simulink model "SimulationDemo_Ship"  (R2025a)
settings: Solver=ode4  StartTime=0.0  StopTime=200  FixedStep=0.02  RelTol=1e-3
InitFcn:
  | Initialization
model workspace (MAT data in the model file):
  actuatorInitial.Aileron_deg = 0
  actuatorInitial.Elevator_deg = 0
  actuatorInitial.Rudder_deg = 0
  contactParams.Kz_Npm = 5000
  contactParams.Cz_Nspm = 160
  contactParams.FrictionMu = 0.03
  contactParams.SlipSpeed_mps = 0.15
  contactParams.RampGain_1pm = 200
  contactParams.NormalScaleMax = 8
  contactParams.GroundPitch_rad = 0.0523598775598
  contactParams.PitchK_NmPerRad = -0.5
  contactParams.PitchC_NmPerRadps = -1
  contactParams.LateralFrictionMu = 1.5
  contactParams.RollK_NmPerRad = -8
  contactParams.RollC_NmPerRadps = -2.5
  contactParams.YawK_NmPerRad = -12
  contactParams.YawC_NmPerRadps = -4
  flightProtection.VMin_mps = 2
  flightProtection.VEps_mps = 0.001
  flightProtection.QGateBreakpoints_mps = [0 2 5]
  flightProtection.QGateTable = [0 0 1]
  flightProtection.BetaGateStartU_mps = 8
  flightProtection.BetaGateFullU_mps = 18
  initial.Heading = -2.35619449019
  initial.Roll = 0
  initial.Pitch = 0.0523598775598
  initial.Yaw = -2.35619449019
  initial.p = 0
  initial.q = 0.0001
  initial.r = 0.0001
  initial.u = 0.1
  initial.v = 0
  initial.w = 0.001
  initial.Altitude_MSL = 0
  initial.Altitude_AGL = 0
  initial.CGInertial.X = 0
  initial.CGInertial.Y = 0
  initial.CGInertial.Z = 0
  initial.Xe = [0 0 0]
  initial.Mass.Empty = 1.67
  initial.Mass.Payload = 1.25
  initial.Mass.GrossTO = 2.92
  initial.Inertia = [0.026  0  0.0007; 0  0.072  0; 0.0007  0  0.096]
undefined symbols (not defined in the file): aeroData, aileronMax, aileronMin, dirPitch, dirRoll, dirThrottle, dirYaw, elevatorMax, elevatorMin, envCatalog, F, geometry, Light, MIL, pitchCh, pitchDB, propulsionData, rollCh, rollDB, rudderMax, rudderMin, throttleCh, throttleDB, uPitchMax, uPitchMin, uRollMax, uRollMin, uThrottleMax, uThrottleMin, uYawMax, uYawMin, yawCh, yawDB
libraries: simulink_extras x4, aerolibwind2 x3, aerolibasang x2, aerolibsim3d x2, aerolibadyn x1, matrix_library x1, aerolibanimutils x1, aerolibatmos2 x1, uavutilslib x1, sim3dlib x1
(part 1 of 2)
settings Model: DataDictionary=environmentData.sldd  Creator=klakhara  LastModifiedBy=klakhara
settings SolverCC: ODENIntegrationMethod=ode4

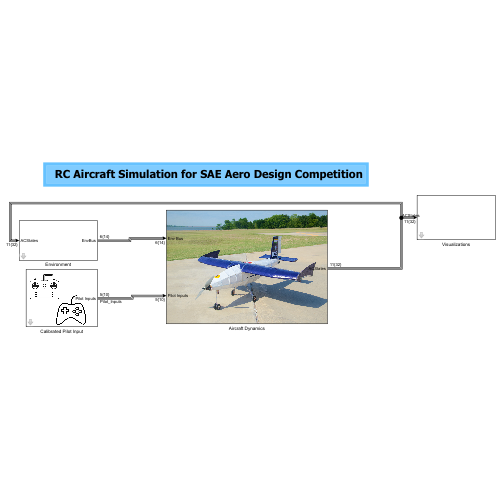
[thumbnail: Simulink's stored preview of the top-level diagram]
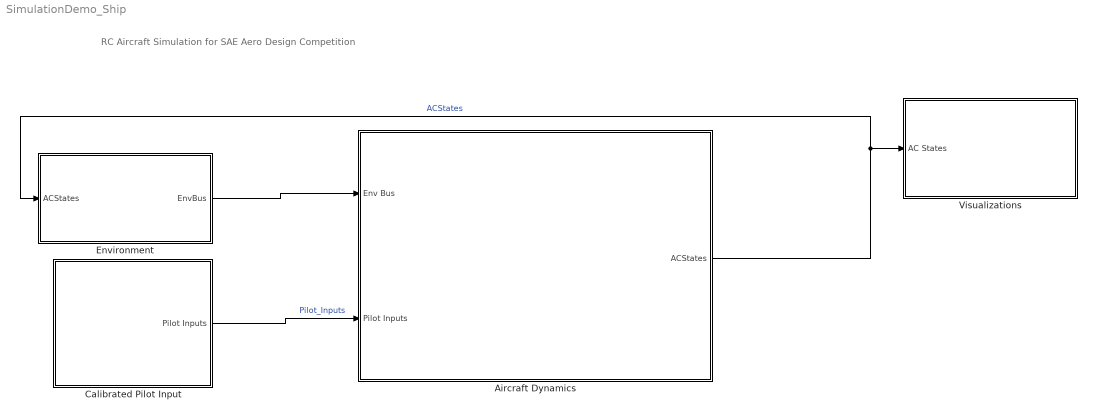
== system SimulationDemo_Ship ==
  note: RC Aircraft Simulation for SAE Aero Design Competition
  Aircraft Dynamics : Subsystem
      mask Display: image('Aircraft.jpg');
  Calibrated Pilot Input : Subsystem  mask{configName=0, joystickID=None}
      mask prompts: joystickID "Device ID:"
      mask TypeOptions joystickID: None | Joystick1 | Joystick2 | Joystick3 | Joystick4 | Joystick5 | Joystick6 | Joystick7 | Joystick8 | Joystick9 | Joystick10 | Joystick11 | Joystick12
      mask DialogControl DescGroupVar Prompt: Import calibration parameters to setup the calibreated input device
      mask DialogControl DescTextVar Prompt: Import your calibration configuration file:
      mask DialogControl loadConfig Prompt: Load file
      mask DialogControl ParameterGroupVar Prompt: Identify your Pilot Input Device:
      mask Display: image('Controller_Setup.jpg');
  Environment : Subsystem  mask{envPreset=Aero Design West — Van Nuys CA (1.1×)}
      mask prompts: envPreset "Select Environment scene"
      mask DialogControl Control1 Prompt: You can select among a variety of environment type along with their difficulty level.
  Visualizations : Subsystem  mask{visualization=Off, FlightParam=on}
      mask prompts: visualization "Trajectory visualization"; FlightParam "Plot flight parameters"
      mask DialogControl DescTextVar Prompt: Select your visualization type and if you want to plot flight paramets in scope.
      mask Display:
      | % Get selected variant from mask
      | v = get_param(gcb, 'visualization');
      | 
      | % Clear icon
      | cla;
      | 
      | 
      | % Choose image based on variant
      | switch v
      |     case '3D Animation'
      |         img = imread('3D_Animation.png');
      |         image(img);
      |         axis off
      |         axis image
      |     case "Unreal Engine"
      |         img = imread('Unreal_Engine.png');
      |         image(img);
      |         axis off
      |         axis image
      |     case 'Off'
      |         % No image
      | 
      | end
      | 
      | % Display image as block icon
  wires:
  Aircraft Dynamics/1(ACStates) -> Environment/1(ACStates), Visualizations/1(AC States)  "ACStates"
  Environment/1(EnvBus) -> Aircraft Dynamics/1(Env Bus)
  Calibrated Pilot Input/1(Pilot Inputs) -> Aircraft Dynamics/2(Pilot Inputs)  "Pilot_Inputs"

== system SimulationDemo_Ship/Aircraft Dynamics ==
  Env Bus : Inport
  Pilot Inputs : Inport  Port=2
  ACStates To Workspace : ToWorkspace  VariableName=ACStates  SaveFormat=Timeseries  SampleTime=-1
  Actuator Dynamics : Subsystem
  Bus Creator : BusCreator  Inputs=8
  Bus Selector : BusSelector  OutputSignals=Actuator deflections
  Equation of motion : EOM6DOFBodyQuat  xme_0=initial.Xe  Vm_0=[initial.u initial.v initial.w]  eul_0=[initial.Roll initial.Pitch initial.Yaw]  pm_0=[initial.p initial.q initial.r]  mass_0=initial.Mass.GrossTO  inertia=initial.Inertia
  Flight Parameters : Subsystem
  Forces & Moments : Subsystem
  Gain : Gain  Gain=[1, 1, -1]
  ACStates : Outport
  wires:
  Actuator Dynamics/1(Actuator_Deflections) -> Bus Creator/8, Forces & Moments/4(Pilot_Inputs)  "Actuator deflections"
  Bus Selector/1 -> Actuator Dynamics/1(Actuator_Command)  "<Actuator deflections>"
  Pilot Inputs/1 -> Bus Selector/1  "Pilot_Inputs"
  Forces & Moments/2(Moments) -> Equation of motion/2
  Forces & Moments/1(Forces) -> Equation of motion/1
  Flight Parameters/1(Flight_Parameters) -> Forces & Moments/2(Flight Params)
  Equation of motion/2 -> Gain/1
  Equation of motion/4 -> Bus Creator/4  "q"
  Gain/1 -> Bus Creator/2  "Xe"
  Env Bus/1 -> Flight Parameters/2(EnvirBus), Forces & Moments/3(Env Bus)
  Equation of motion/1 -> Bus Creator/1  "Ve"
  Equation of motion/5 -> Bus Creator/5  "DCM_be"
  Equation of motion/7 -> Bus Creator/7  "wb"
  Equation of motion/6 -> Bus Creator/6  "Vb"
  Equation of motion/3 -> Bus Creator/3  "Euler_angles"
  Bus Creator/1 -> Forces & Moments/1(States), Flight Parameters/1("AC States "), ACStates To Workspace/1, ACStates/1  "ACStates"

== system SimulationDemo_Ship/Calibrated Pilot Input ==
  Actuator scaling : Subsystem
  Bus Creator : BusCreator  Inputs=2
  Pilot Joystick All : aerolibanimutils/Pilot Joystick  JoystickID=None  OutputConfiguration=AllOutputs  SampleTime=0.5
  PilotInput : BusCreator  Inputs=4
  Terminator : Terminator
  Terminator1 : Terminator
  Pilot Inputs : Outport
  wires:
  Bus Creator/1 -> Pilot Inputs/1
  Pilot Joystick All/1 -> Bus Creator/1, Actuator scaling/1(In1)  "Raw Inputs"
  Actuator scaling/2(Elevator) -> PilotInput/2  "Elevator"
  Pilot Joystick All/2 -> Terminator/1
  PilotInput/1 -> Bus Creator/2  "Actuator deflections"
  Actuator scaling/3(Rudder) -> PilotInput/3  "Rudder"
  Actuator scaling/4(Throttle) -> PilotInput/4  "Throttle"
  Actuator scaling/1(Aileron) -> PilotInput/1  "Aileron"
  Pilot Joystick All/3 -> Terminator1/1

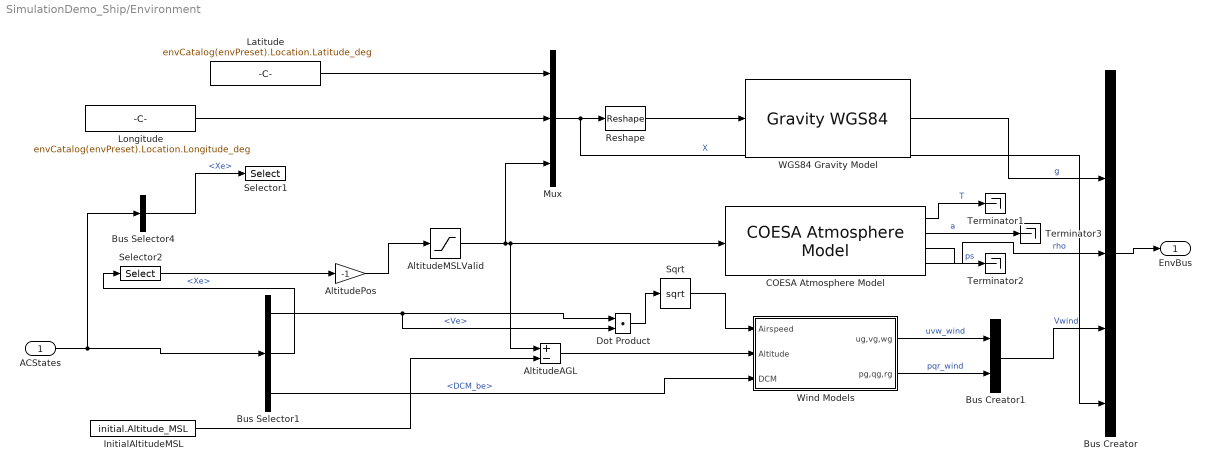
== system SimulationDemo_Ship/Environment ==
  ACStates : Inport
  AltitudeAGL : Sum  Inputs=+-
  AltitudeMSLValid : Saturate  UpperLimit=84852  LowerLimit=0
  AltitudePos : Gain  Gain=-1
  Bus Creator : BusCreator  Inputs=5
  Bus Creator1 : BusCreator  Inputs=2
  Bus Selector1 : BusSelector  OutputSignals=Ve,Xe,DCM_be
  Bus Selector4 : BusSelector  OutputSignals=Xe
  COESA Atmosphere Model : aerolibatmos2/COESA Atmosphere Model  units=Metric (MKS)  spec=1976 COESA-extended U.S. Standard Atmosphere  model=Profile  profile_var=High temperature  profile_percent=1%  profile_alt=5 km (16404 ft)  envelope_var=High temperature  envelope_percent=1%  action=Warning
  Dot Product : DotProduct  OutDataTypeStr=Inherit: Inherit via internal rule
  InitialAltitudeMSL : Constant  Value=initial.Altitude_MSL
  "Latitude " : Constant  Value=envCatalog(envPreset).Location.Latitude_deg
  Longitude : Constant  Value=envCatalog(envPreset).Location.Longitude_deg
  Mux : Mux  Inputs=3
  Reshape : Reshape  OutputDimensionality=Row vector (2-D)
  Selector1 : Selector  IndexMode=Zero-based  InputPortWidth=3  IndexOptions=Index vector (dialog)  Indices=2  OutputSizes=1
  Selector2 : Selector  IndexMode=Zero-based  InputPortWidth=3  IndexOptions=Index vector (dialog)  Indices=2  OutputSizes=1
  Sqrt : Sqrt
  Terminator1 : Terminator
  Terminator2 : Terminator
  Terminator3 : Terminator
  "WGS84 Gravity Model  " : GravityWGS84  action=None
  Wind Models : Subsystem
  EnvBus : Outport  VectorParamsAs1DForOutWhenUnconnected=off
  wires:
  AltitudeMSLValid/1 -> COESA Atmosphere Model/1, AltitudeAGL/1, Mux/3
  AltitudePos/1 -> AltitudeMSLValid/1
  AltitudeAGL/1 -> Wind Models/2(Altitude)
  InitialAltitudeMSL/1 -> AltitudeAGL/2
  Selector2/1 -> AltitudePos/1
  Bus Selector1/2 -> Selector2/1  "<Xe>"
  Bus Selector1/3 -> Wind Models/3(DCM)  "<DCM_be>"
  Reshape/1 -> "WGS84 Gravity Model  "/1
  "WGS84 Gravity Model  "/1 -> Bus Creator/2  "g"
  Mux/1 -> Reshape/1, Bus Creator/5  "X"
  Longitude/1 -> Mux/2
  "Latitude "/1 -> Mux/1
  Bus Selector1/1 -> Dot Product/1, Dot Product/2  "<Ve>"
  ACStates/1 -> Bus Selector4/1, Bus Selector1/1
  Bus Selector4/1 -> Selector1/1  "<Xe>"
  Bus Creator/1 -> EnvBus/1
  Sqrt/1 -> Wind Models/1(Airspeed)
  Dot Product/1 -> Sqrt/1
  Bus Creator1/1 -> Bus Creator/4  "Vwind"
  Wind Models/1(ug,vg,wg) -> Bus Creator1/1  "uvw_wind"
  Wind Models/2(pg,qg,rg) -> Bus Creator1/2  "pqr_wind"
  COESA Atmosphere Model/2 -> Terminator3/1  "a"
  COESA Atmosphere Model/3 -> Terminator2/1  "ps"
  COESA Atmosphere Model/1 -> Terminator1/1  "T"
  COESA Atmosphere Model/4 -> Bus Creator/3  "rho"

== system SimulationDemo_Ship/Visualizations ==
  AC States : Inport
  "Flight parameters " : Subsystem  Variant=on  EmptyChoice=on
  Trajectory Visualization : Subsystem  Variant=on  EmptyChoice=on
  wires:
  AC States/1 -> Trajectory Visualization/1(AC States), "Flight parameters "/1(In1)

== system SimulationDemo_Ship/Aircraft Dynamics/Actuator Dynamics ==
  Actuator_Command : Inport
  Aileron_Command_Limit : Saturate  UpperLimit=geometry.AileronLimit(2)  LowerLimit=geometry.AileronLimit(1)
  Aileron_Deflection_Limit : Saturate  UpperLimit=geometry.AileronLimit(2)  LowerLimit=geometry.AileronLimit(1)
  Aileron_Lag_0p05s : StateSpace  A=-20  B=20  D=0  InitialCondition=actuatorInitial.Aileron_deg
  Aileron_Rate_300dps : RateLimiter  RisingSlewLimit=300  FallingSlewLimit=-300  InitialCondition=actuatorInitial.Aileron_deg
  Command_Select : BusSelector  OutputSignals=Aileron,Elevator,Rudder,Throttle
  Deflection_Bus : BusCreator  Inputs=4
  Elevator_Command_Limit : Saturate  UpperLimit=geometry.ElevatorLimit(2)  LowerLimit=geometry.ElevatorLimit(1)
  Elevator_Deflection_Limit : Saturate  UpperLimit=geometry.ElevatorLimit(2)  LowerLimit=geometry.ElevatorLimit(1)
  Elevator_Lag_0p05s : StateSpace  A=-20  B=20  D=0  InitialCondition=actuatorInitial.Elevator_deg
  Elevator_Rate_300dps : RateLimiter  RisingSlewLimit=300  FallingSlewLimit=-300  InitialCondition=actuatorInitial.Elevator_deg
  Rudder_Command_Limit : Saturate  UpperLimit=geometry.RudderLimit(2)  LowerLimit=geometry.RudderLimit(1)
  Rudder_Deflection_Limit : Saturate  UpperLimit=geometry.RudderLimit(2)  LowerLimit=geometry.RudderLimit(1)
  Rudder_Lag_0p05s : StateSpace  A=-20  B=20  D=0  InitialCondition=actuatorInitial.Rudder_deg
  Rudder_Rate_300dps : RateLimiter  RisingSlewLimit=300  FallingSlewLimit=-300  InitialCondition=actuatorInitial.Rudder_deg
  Actuator_Deflections : Outport
  wires:
  Actuator_Command/1 -> Command_Select/1
  Aileron_Command_Limit/1 -> Aileron_Lag_0p05s/1
  Command_Select/1 -> Aileron_Command_Limit/1  "<Aileron>"
  Command_Select/2 -> Elevator_Command_Limit/1  "<Elevator>"
  Command_Select/3 -> Rudder_Command_Limit/1  "<Rudder>"
  Elevator_Command_Limit/1 -> Elevator_Lag_0p05s/1
  Command_Select/4 -> Deflection_Bus/4  "<Throttle>"
  Rudder_Command_Limit/1 -> Rudder_Lag_0p05s/1
  Aileron_Lag_0p05s/1 -> Aileron_Rate_300dps/1
  Elevator_Lag_0p05s/1 -> Elevator_Rate_300dps/1
  Rudder_Lag_0p05s/1 -> Rudder_Rate_300dps/1
  Aileron_Rate_300dps/1 -> Aileron_Deflection_Limit/1
  Elevator_Rate_300dps/1 -> Elevator_Deflection_Limit/1
  Rudder_Rate_300dps/1 -> Rudder_Deflection_Limit/1
  Elevator_Deflection_Limit/1 -> Deflection_Bus/2  "Elevator"
  Aileron_Deflection_Limit/1 -> Deflection_Bus/1  "Aileron"
  Rudder_Deflection_Limit/1 -> Deflection_Bus/3  "Rudder"
  Deflection_Bus/1 -> Actuator_Deflections/1

== system SimulationDemo_Ship/Aircraft Dynamics/Flight Parameters ==
  "AC States " : Inport
  EnvirBus : Inport  Port=2
  Bus Creator : BusCreator  Inputs=6
  Bus Selector1 : BusSelector  OutputSignals=rho
  Bus Selector2 : BusSelector  OutputSignals=Vb
  Bus Selector3 : BusSelector  OutputSignals=wb
  Bus Selector4 : BusSelector  OutputSignals=Vwind.uvw_wind,Vwind.pqr_wind
  Flight Parameters To Workspace : ToWorkspace  VariableName=FlightParameters  SaveFormat=Timeseries  SampleTime=-1
  "Incidence, Sideslip, & Airspeed" : aerolibasang/Incidence, Sideslip, & Airspeed
  Radians to Degrees : simulink_extras/Transformations/Radians to Degrees
  Radians to Degrees1 : simulink_extras/Transformations/Radians to Degrees
  Subsystem : Subsystem
      settings: PortSchema="{\"entries\":[{\"content\":{\"sides\":[{\"content\":{\"connectorIds\":[\"In1\",\"In2\"]},\"type\":\"ConnectorPlacement.EquallySpacedRectSide\",\"uuid\":\"5a143d0f-2436-4fb0-bb97-2c4984d07975\"},{\"content\":{\"connectorIds\":[\"Out1\"],\"side\":\"RIGHT\"},\"type\":\"ConnectorPlacement.EquallySpacedRectSide\",\"uuid\":\"8d58a2ee-82c7-4615-9bab-8cc4c0d46ad5\"},{\"content\":{\"connectorIds\":[\"In3\"],\"side\":\"TOP\"},\"type\":\"ConnectorPlacement.EquallySpacedRectSide\",\"uuid\":\"18f756c1-07a2-4df5-83f0-d5c22876817a\"}]},\"type\":\"ConnectorPlacement.EquallySpacedConnector\",\"uuid\":\"42d60932-45cf-443a-a7ca-3ff9305e2569\"}],\"packageUris\":[\"http://schema.mathworks.com/mf0/Connector/R2020b\"],\"version\":\"1.0\"}"
  Sum2 : Sum  InputSameDT=on  SaturateOnIntegerOverflow=on  OutDataTypeStr=Inherit: Same as first input
  Sum4 : Sum  Inputs=+-|  InputSameDT=on  SaturateOnIntegerOverflow=on  OutDataTypeStr=Inherit: Same as first input
  Vrel_safe : Subsystem
  Flight_Parameters : Outport  VectorParamsAs1DForOutWhenUnconnected=off
  wires:
  "AC States "/1 -> Bus Selector2/1, Bus Selector3/1
  Sum2/1 -> Bus Creator/5  "pqr_tot"
  Sum4/1 -> Vrel_safe/1(Vrel)  "Vrel"
  Bus Selector3/1 -> Sum2/2  "<wb>"
  EnvirBus/1 -> Bus Selector1/1, Bus Selector4/1
  Bus Selector2/1 -> Sum4/1  "<Vb>"
  Bus Selector4/2 -> Sum2/1  "<pqr_wind>"
  Bus Selector4/1 -> Sum4/2  "<uvw_wind>"
  "Incidence, Sideslip, & Airspeed"/3 -> Subsystem/3(TAS), Bus Creator/4  "TAS"
  "Incidence, Sideslip, & Airspeed"/1 -> Radians to Degrees/1
  "Incidence, Sideslip, & Airspeed"/2 -> Radians to Degrees1/1
  Vrel_safe/1(Vrel_safe) -> Subsystem/1(Vrel_safe), "Incidence, Sideslip, & Airspeed"/1, Bus Creator/1  "Vrel"
  Bus Selector1/1 -> Subsystem/2(<rho>)  "<rho>"
  Subsystem/1(q) -> Bus Creator/6  "dynamic Pressure"
  Radians to Degrees/1 -> Bus Creator/2  "alpha"
  Radians to Degrees1/1 -> Bus Creator/3  "beta"
  Bus Creator/1 -> Flight Parameters To Workspace/1, Flight_Parameters/1

== system SimulationDemo_Ship/Aircraft Dynamics/Forces & Moments ==
  note: Forces & Moments
      | 1. Gravitational Forces
      | 2. Aerodynamic Forces & Moments
      | 3. Propulsion Forces & Moments
  States : Inport
  Flight Params : Inport  Port=2
  Env Bus : Inport  Port=3
  Pilot_Inputs : Inport  Port=4
  Aerodynamic Forces & Moments : Subsystem
  Bus Selector : BusSelector  OutputSignals=g
  Bus Selector1 : BusSelector  OutputSignals=Xe,DCM_be,Vb
  Contact Forces & Moments : Subsystem
  Gravitational Forces : Subsystem
  Propulsion Forces & Moments : Subsystem
  Sum : Sum  Inputs=++++
  Sum1 : Sum  Inputs=+++
  Forces : Outport
  Moments : Outport  Port=2
  wires:
  Bus Selector1/3 -> Contact Forces & Moments/4(Vb)  "<Vb>"
  Contact Forces & Moments/1(F_Contact) -> Sum/4
  Bus Selector1/1 -> Contact Forces & Moments/2(Xe)  "<Xe>"
  Bus Selector1/2 -> Gravitational Forces/1(DCM)  "<DCM_be>"
  Sum1/1 -> Moments/1  "Moments"
  Sum/1 -> Forces/1  "Forces"
  Propulsion Forces & Moments/1(Forces_Propulsion) -> Sum/3  "F_Prop"
  Aerodynamic Forces & Moments/1(Forces_aero) -> Sum/2  "F_Aero"
  Gravitational Forces/1(Fgrav) -> Sum/1, Contact Forces & Moments/3(F_Gravity)  "F_Gravity"
  Bus Selector/1 -> Gravitational Forces/2(g)  "<g>"
  States/1 -> Bus Selector1/1, Contact Forces & Moments/1(States)  "States"
  Env Bus/1 -> Propulsion Forces & Moments/2(EnvBus), Bus Selector/1
  Flight Params/1 -> Aerodynamic Forces & Moments/1(Flight Params)
  Propulsion Forces & Moments/2(Moments_Propulsion) -> Sum1/2  "M_Prop"
  Pilot_Inputs/1 -> Aerodynamic Forces & Moments/2(Pilot_Input), Propulsion Forces & Moments/1(Pilot Inputs)
  Aerodynamic Forces & Moments/2(Moments_aero) -> Sum1/1  "M_Aero"
  Contact Forces & Moments/2(M_Contact) -> Sum1/3  "M_Contact"

== system SimulationDemo_Ship/Calibrated Pilot Input/Actuator scaling ==
  In1 : Inport
  Aileron Scaling : Subsystem
  Demux : Demux
  Elevator Scaling : Subsystem
  Rudder Scaling : Subsystem
  Selector : Selector  InputPortWidth=6  IndexOptions=Index vector (dialog)  Indices=[rollCh pitchCh yawCh throttleCh]  OutputSizes=1
  Throttle Scaling : Subsystem
  Aileron : Outport
  Elevator : Outport  Port=2
  Rudder : Outport  Port=3
  Throttle : Outport  Port=4
  wires:
  In1/1 -> Selector/1
  Rudder Scaling/1(actuator deflection) -> Rudder/1
  Demux/3 -> Rudder Scaling/1(raw signal)  "Yaw"
  Demux/1 -> Aileron Scaling/1(raw signal)  "roll"
  Elevator Scaling/1(actuator deflection) -> Elevator/1
  Demux/4 -> Throttle Scaling/1(raw signal)  "Throttle"
  Demux/2 -> Elevator Scaling/1(raw signal)  "Pitch"
  Aileron Scaling/1(actuator deflection) -> Aileron/1
  Throttle Scaling/1(actuator deflection) -> Throttle/1
  Selector/1 -> Demux/1

== system SimulationDemo_Ship/Environment/Wind Models ==
  Airspeed : Inport  Unit=m/s
  Altitude : Inport  Port=2  Unit=meter
  DCM : Inport  Port=3
  "DCM " : InportShadow  Port=3
  Discrete Wind Gust Model : aerolibwind2/Discrete Wind Gust Model  units=Metric (MKS)  Gx=off  Gy=off  Gz=off  t_0=envCatalog(envPreset).Gust.StartTime_s  d_m=envCatalog(envPreset).Gust.Length_m  v_m=envCatalog(envPreset).Gust.Amplitude_mps
  Dryden Wind Turbulence Model (Continuous (+q -r)) : aerolibwind2/Dryden Wind Turbulence Model  (Continuous (+q -r))  units=Metric (MKS)  spec=MIL-F-8785C  model=Continuous Dryden (+q -r)  W20=envCatalog(envPreset).Turbulence.Speed_6m_mps  Wdeg=envCatalog(envPreset).Turbulence.Direction_deg  TurbProb=10^-2 - Light  L_high=envCatalog(envPreset).Turbulence.Scale_Lu_m  Wingspan=geometry.Area  ts=0.5  Seed=envCatalog(envPreset).Turbulence.NoiseSeeds  T_on=off
  Sum : Sum  Inputs=+++  InputSameDT=on  SaturateOnIntegerOverflow=on  OutDataTypeStr=Inherit: Same as first input
  Wind Shear Model : aerolibwind2/Wind Shear Model  units=Metric (MKS)  phase=Category C - Terminal Flight Phase  W_20=envCatalog(envPreset).WindShear.Speed_6m_mps  Wdeg=envCatalog(envPreset).WindShear.Direction_deg
  ug,vg,wg : Outport  Unit=m/s  VectorParamsAs1DForOutWhenUnconnected=off
  pg,qg,rg : Outport  Port=2  Unit=rad/second  VectorParamsAs1DForOutWhenUnconnected=off
  wires:
  "DCM "/1 -> Dryden Wind Turbulence Model (Continuous (+q -r))/3
  Wind Shear Model/1 -> Sum/1
  Dryden Wind Turbulence Model (Continuous (+q -r))/1 -> Sum/2
  Discrete Wind Gust Model/1 -> Sum/3
  Sum/1 -> ug,vg,wg/1
  DCM/1 -> Wind Shear Model/2
  Airspeed/1 -> Dryden Wind Turbulence Model (Continuous (+q -r))/2, Discrete Wind Gust Model/1
  Dryden Wind Turbulence Model (Continuous (+q -r))/2 -> pg,qg,rg/1
  Altitude/1 -> Dryden Wind Turbulence Model (Continuous (+q -r))/1, Wind Shear Model/1

== system SimulationDemo_Ship/Visualizations/Flight parameters  ==
  In1 : Inport
  Scope Plot : Subsystem  TreatAsAtomicUnit=on  VariantControl=FlightParam ==1

== system SimulationDemo_Ship/Visualizations/Trajectory Visualization ==
  AC States : Inport
  3D Animation : Subsystem  VariantControl="visualization == \"3D Animation\""
      mask Display: image('3D_Animation.png');
  Unreal Engine : Subsystem  VariantControl="visualization == \"Unreal Engine\""
      mask Display: image('Unreal_Engine.png');

== system SimulationDemo_Ship/Aircraft Dynamics/Flight Parameters/Subsystem ==
  note: Note: 1D lookup table here is used as a switch to protect dynamic pressure for speed below 2 m/sec and gradually ramps up till 5 m/sec.
  Vrel_safe : Inport
  <rho> : Inport  Port=2
  TAS : Inport  Port=3
  1-D Lookup Table : Lookup_n-D  NumberOfTableDimensions=1  BreakpointsForDimension1=flightProtection.QGateBreakpoints_mps  Table=flightProtection.QGateTable  InterpMethod=Flat  ExtrapMethod=Clip  InternalRulePriority=Speed  RndMeth=Simplest
  Dynamic Pressure : aerolibasang/Dynamic Pressure
  Product : Product
  q : Outport
  wires:
  Vrel_safe/1 -> Dynamic Pressure/1
  <rho>/1 -> Dynamic Pressure/2
  1-D Lookup Table/1 -> Product/1
  Dynamic Pressure/1 -> Product/2
  Product/1 -> q/1
  TAS/1 -> 1-D Lookup Table/1

== system SimulationDemo_Ship/Aircraft Dynamics/Flight Parameters/Vrel_safe ==
  Vrel : Inport
  Mux_Vrel_safe : Mux  Inputs=3
  Split_Vrel : Demux  Outputs=3
  V_denom : MinMax  Function=max  Inputs=2
  V_min : Constant  Value=flightProtection.VMin_mps
  V_safe : MinMax  Function=max  Inputs=2
  eps_V : Constant  Value=flightProtection.VEps_mps
  scale : Product  Inputs=*/
  speed_sq : Sum  Inputs=+++
  sqrt_speed : Math  Operator=sqrt  SignedPower=on  RndMeth=Zero
  u_safe : Product
  u_sq : Product
  v_safe : Product
  v_sq : Product
  w_safe : Product
  w_sq : Product
  Vrel_safe : Outport
  wires:
  speed_sq/1 -> sqrt_speed/1  "V_mag_sq"
  Vrel/1 -> Split_Vrel/1
  u_sq/1 -> speed_sq/1
  w_sq/1 -> speed_sq/3
  Split_Vrel/1 -> u_sq/2, u_sq/1, u_safe/1  "u_rel"
  Split_Vrel/2 -> v_sq/1, v_sq/2, v_safe/1  "v_rel"
  v_sq/1 -> speed_sq/2
  Split_Vrel/3 -> w_safe/1, w_sq/2, w_sq/1  "w_rel"
  V_min/1 -> V_safe/2
  sqrt_speed/1 -> V_safe/1, V_denom/1  "V_mag"
  eps_V/1 -> V_denom/2
  V_safe/1 -> scale/1  "V_safe_mag"
  V_denom/1 -> scale/2
  u_safe/1 -> Mux_Vrel_safe/1  "u_rel_safe"
  scale/1 -> v_safe/2, w_safe/2, u_safe/2  "V_guard_scale"
  w_safe/1 -> Mux_Vrel_safe/3  "w_rel_safe"
  v_safe/1 -> Mux_Vrel_safe/2  "v_rel_safe"
  Mux_Vrel_safe/1 -> Vrel_safe/1  "Vrel_safe"

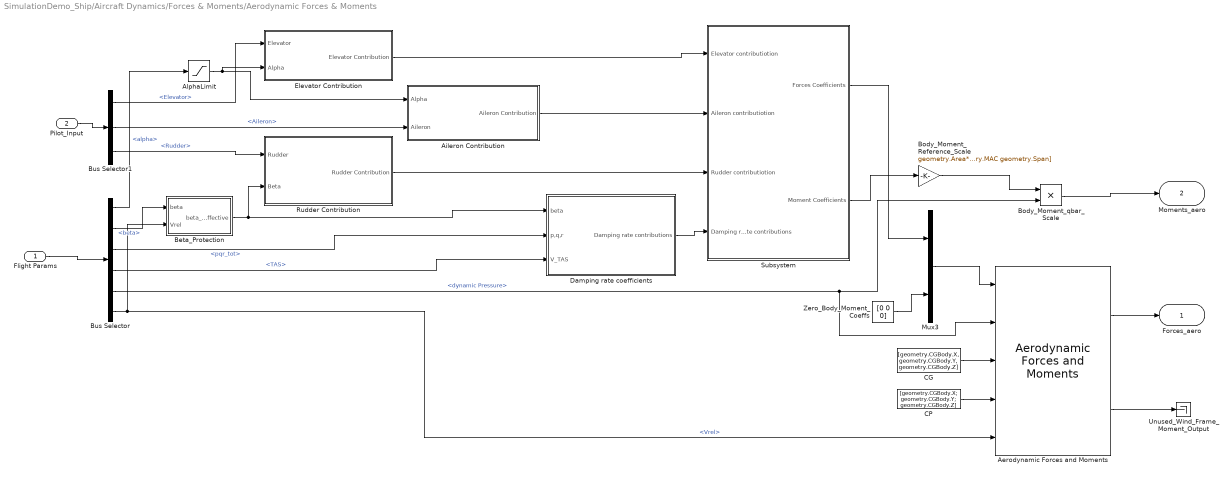
== system SimulationDemo_Ship/Aircraft Dynamics/Forces & Moments/Aerodynamic Forces & Moments ==
  Flight Params : Inport
  Pilot_Input : Inport  Port=2
  "Aerodynamic Forces and Moments " : aerolibadyn/Aerodynamic Forces and Moments   inputAxes=Wind  outputForceAxes=Body  outputMomentAxes=Body  S=geometry.Area  b=geometry.Span  cbar=geometry.MAC
  Aileron Contribution : Subsystem
  AlphaLimit : Saturate  UpperLimit=aeroData.validAlphaRange_deg(2)  LowerLimit=aeroData.validAlphaRange_deg(1)
  Beta_Protection : Subsystem
  Body_Moment_Reference_Scale : Gain  Gain=geometry.Area*[geometry.Span geometry.MAC geometry.Span]
  Body_Moment_qbar_Scale : Product
  Bus Selector : BusSelector  OutputSignals=alpha,beta,pqr_tot,TAS,dynamic Pressure,Vrel
  Bus Selector1 : BusSelector  OutputSignals=Elevator,Aileron,Rudder
  CG : Constant  Value="[geometry.CGBody.X, geometry.CGBody.Y,  geometry.CGBody.Z]"
  CP : Constant  Value=[geometry.CGBody.X; geometry.CGBody.Y; geometry.CGBody.Z]
  Damping rate coefficients : Subsystem
  Elevator Contribution : Subsystem
  Mux3 : Mux  Inputs=2
  Rudder Contribution : Subsystem
  Subsystem : Subsystem
  Unused_Wind_Frame_Moment_Output : Terminator
  Zero_Body_Moment_Coeffs : Constant  Value=[0 0 0]
  Forces_aero : Outport
  Moments_aero : Outport  Port=2
  wires:
  "Aerodynamic Forces and Moments "/2 -> Unused_Wind_Frame_Moment_Output/1
  Bus Selector/1 -> AlphaLimit/1  "<alpha>"
  Flight Params/1 -> Bus Selector/1
  Bus Selector/4 -> Damping rate coefficients/3(V_TAS)  "<TAS>"
  AlphaLimit/1 -> Elevator Contribution/2(Alpha), Aileron Contribution/1(Alpha)
  Bus Selector/2 -> Beta_Protection/1(beta)  "<beta>"
  Bus Selector/3 -> Damping rate coefficients/2(p,q,r)  "<pqr_tot>"
  Elevator Contribution/1(Elevator Contribution) -> Subsystem/1(Elevator contributiotion)
  Bus Selector/5 -> Body_Moment_qbar_Scale/2, "Aerodynamic Forces and Moments "/2  "<dynamic Pressure>"
  Bus Selector/6 -> Beta_Protection/2(Vrel), "Aerodynamic Forces and Moments "/5  "<Vrel>"
  CG/1 -> "Aerodynamic Forces and Moments "/3
  CP/1 -> "Aerodynamic Forces and Moments "/4
  Pilot_Input/1 -> Bus Selector1/1
  Bus Selector1/1 -> Elevator Contribution/1(Elevator)  "<Elevator>"
  Bus Selector1/2 -> Aileron Contribution/2(Aileron)  "<Aileron>"
  Bus Selector1/3 -> Rudder Contribution/1(Rudder)  "<Rudder>"
  Aileron Contribution/1(Aileron Contribution) -> Subsystem/2(Aileron contributiotion)
  Rudder Contribution/1("Rudder Contribution ") -> Subsystem/3(Rudder contributiotion)
  Damping rate coefficients/1(Damping rate contributions) -> Subsystem/4(Damping rate contributions)
  Subsystem/1(Forces Coefficients) -> Mux3/1
  Mux3/1 -> "Aerodynamic Forces and Moments "/1
  "Aerodynamic Forces and Moments "/1 -> Forces_aero/1
  Beta_Protection/1(beta_effective) -> Damping rate coefficients/1(beta), Rudder Contribution/2(Beta)
  Zero_Body_Moment_Coeffs/1 -> Mux3/2
  Subsystem/2(Moment Coefficients) -> Body_Moment_Reference_Scale/1
  Body_Moment_Reference_Scale/1 -> Body_Moment_qbar_Scale/1
  Body_Moment_qbar_Scale/1 -> Moments_aero/1

== system SimulationDemo_Ship/Aircraft Dynamics/Forces & Moments/Contact Forces & Moments ==
  States : Inport
  Xe : Inport  Port=2
  F_Gravity : Inport  Port=3
  Vb : Inport  Port=4
  Contact_Force_Total : Sum
  Ground_Contact_Switch : Switch  Criteria=u2 > Threshold  Threshold=initial.Mass.GrossTO*9.80665/contactParams.Kz_Npm
  Normal_Friction_Forces : Subsystem
  Pitch_Contact_Moment : Subsystem
  Select_Ze : Selector  InputPortWidth=3  IndexOptions=Index vector (dialog)  Indices=[3]  OutputSizes=1
  Zero_Force : Constant  Value=[0;0;0]
  F_Contact : Outport
  M_Contact : Outport  Port=2
  wires:
  Pitch_Contact_Moment/1(M_Contact) -> M_Contact/1  "M_Contact"
  States/1 -> Normal_Friction_Forces/4(States), Pitch_Contact_Moment/1(States)
  Normal_Friction_Forces/2(F_Contact_Friction) -> Contact_Force_Total/2
  Normal_Friction_Forces/1(F_Contact_Normal) -> Contact_Force_Total/1
  Vb/1 -> Normal_Friction_Forces/3(Vb)
  F_Gravity/1 -> Normal_Friction_Forces/2(F_Gravity)
  Contact_Force_Total/1 -> Ground_Contact_Switch/3
  Ground_Contact_Switch/1 -> F_Contact/1
  Zero_Force/1 -> Ground_Contact_Switch/1
  Select_Ze/1 -> Normal_Friction_Forces/1(Ze), Ground_Contact_Switch/2
  Xe/1 -> Select_Ze/1

== system SimulationDemo_Ship/Aircraft Dynamics/Forces & Moments/Gravitational Forces ==
  DCM : Inport
  g : Inport  Port=2  Unit=m/s^2
  Gross TO mass : Gain  Gain=initial.Mass.GrossTO  SaturateOnIntegerOverflow=on  OutDataTypeStr=Inherit: Same as input  ParamDataTypeStr=Inherit: Same as input
  Inertial to Body : Product  Multiplication=Matrix(*)  InputSameDT=on  SaturateOnIntegerOverflow=on  OutDataTypeStr=Inherit: Same as first input
  Reshape : Reshape  OutputDimensionality=Column vector (2-D)
  Reshape1 : Reshape
  Fgrav : Outport  Unit=N  VectorParamsAs1DForOutWhenUnconnected=off
  wires:
  Inertial to Body/1 -> Reshape1/1
  g/1 -> Gross TO mass/1
  DCM/1 -> Inertial to Body/1
  Gross TO mass/1 -> Reshape/1
  Reshape/1 -> Inertial to Body/2
  Reshape1/1 -> Fgrav/1

== system SimulationDemo_Ship/Aircraft Dynamics/Forces & Moments/Propulsion Forces & Moments ==
  Pilot Inputs : Inport
  EnvBus : Inport  Port=2
  Density Correction : Subsystem
  Gain : Gain
  Product : Product
  Subsystem : Subsystem
      settings: PortSchema="{\"entries\":[{\"content\":{\"sides\":[{\"content\":{\"connectorIds\":[\"Out1\"]},\"type\":\"ConnectorPlacement.EquallySpacedRectSide\",\"uuid\":\"fb30b856-b505-4c52-9be5-f51b9b4f9b3d\"},{\"content\":{\"side\":\"RIGHT\"},\"type\":\"ConnectorPlacement.EquallySpacedRectSide\",\"uuid\":\"6b49ea0c-e042-48c7-9a23-d0c81f552445\"},{\"content\":{\"connectorIds\":[\"In1\"],\"side\":\"TOP\"},\"type\":\"ConnectorPlacement.EquallySpacedRectSide\",\"uuid\":\"9dc7e958-cdfa-43a2-9a4f-607dc953e274\"}]},\"type\":\"ConnectorPlacement.EquallySpacedConnector\",\"uuid\":\"2adf19d2-e141-4d29-811e-0d4bf7e85bad\"}],\"packageUris\":[\"http://schema.mathworks.com/mf0/Connector/R2020b\"],\"version\":\"1.0\"}"
  Subsystem1 : Subsystem
  Subsystem2 : Subsystem
  Forces_Propulsion : Outport
  Moments_Propulsion : Outport  Port=2
  wires:
  Gain/1 -> Forces_Propulsion/1, Subsystem/1(Forces)
  Product/1 -> Subsystem1/1(Density corrected Thrust)
  Subsystem1/1(Forces_Propulsion) -> Gain/1
  Subsystem/1(Moments) -> Moments_Propulsion/1  "Moments_Propulsion"
  EnvBus/1 -> Density Correction/1(In1)
  Density Correction/1(Out1) -> Product/2
  Pilot Inputs/1 -> Subsystem2/1(Pilot_Inputs)  "Pilot_Inputs"
  Subsystem2/1(Motor_Prop_Thrust) -> Product/1

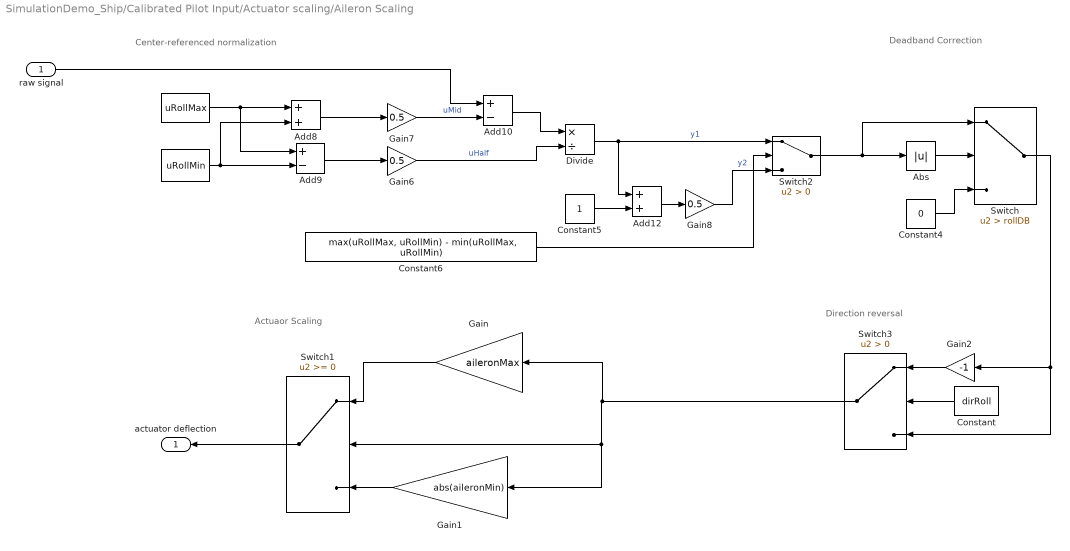
== system SimulationDemo_Ship/Calibrated Pilot Input/Actuator scaling/Aileron Scaling ==
  note: Direction reversal
  note: Center-referenced normalization
  note: Deadband Correction
  note: Actuaor Scaling
  raw signal : Inport
  " " : Constant  Value=uRollMin
  "   " : Constant  Value=uRollMax
  Abs : Abs  SaturateOnIntegerOverflow=off
  Add10 : Sum  Inputs=+-
  Add12 : Sum
  Add8 : Sum
  Add9 : Sum  Inputs=+-
  Constant : Constant  Value=dirRoll
  Constant4 : Constant  Value=0
  Constant5 : Constant
  Constant6 : Constant  Value=max(uRollMax, uRollMin) - min(uRollMax, uRollMin)
  Divide : Product  Inputs=*/
  Gain : Gain  Gain=aileronMax
  Gain1 : Gain  Gain=abs(aileronMin)
  Gain2 : Gain  Gain=-1
  Gain6 : Gain  Gain=0.5
  Gain7 : Gain  Gain=0.5
  Gain8 : Gain  Gain=0.5
  Switch : Switch  Criteria=u2 > Threshold  Threshold=rollDB  SaturateOnIntegerOverflow=off  InputSameDT=off
  Switch1 : Switch  SaturateOnIntegerOverflow=off  InputSameDT=off
  Switch2 : Switch  Criteria=u2 > Threshold  SaturateOnIntegerOverflow=off  InputSameDT=off
  Switch3 : Switch  Criteria=u2 > Threshold  SaturateOnIntegerOverflow=off  InputSameDT=off
  actuator deflection : Outport
  wires:
  Add9/1 -> Gain6/1
  "   "/1 -> Add9/1, Add8/1
  Add8/1 -> Gain7/1
  " "/1 -> Add8/2, Add9/2
  raw signal/1 -> Add10/1
  Gain7/1 -> Add10/2  "uMid"
  Add10/1 -> Divide/1
  Gain6/1 -> Divide/2  "uHalf"
  Switch1/1 -> actuator deflection/1
  Divide/1 -> Add12/1, Switch2/1  "y1"
  Constant5/1 -> Add12/2
  Add12/1 -> Gain8/1
  Constant6/1 -> Switch2/2
  Gain8/1 -> Switch2/3  "y2"
  Abs/1 -> Switch/2
  Constant4/1 -> Switch/3
  Switch/1 -> Gain2/1, Switch3/3
  Gain/1 -> Switch1/1
  Gain1/1 -> Switch1/3
  Gain2/1 -> Switch3/1
  Switch3/1 -> Gain1/1, Switch1/2, Gain/1
  Constant/1 -> Switch3/2
  Switch2/1 -> Switch/1, Abs/1

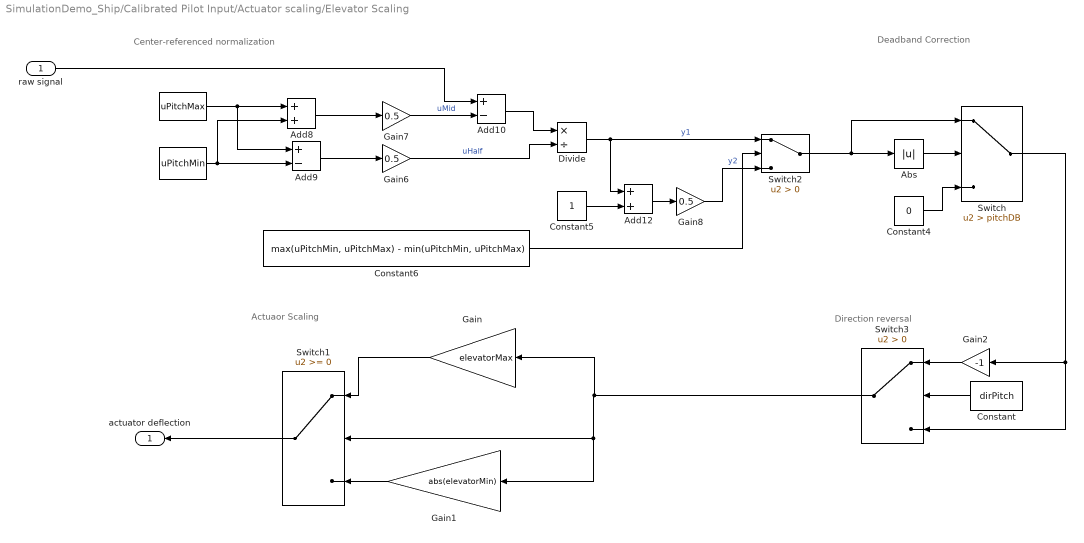
== system SimulationDemo_Ship/Calibrated Pilot Input/Actuator scaling/Elevator Scaling ==
  note: Direction reversal
  note: Center-referenced normalization
  note: Deadband Correction
  note: Actuaor Scaling
  raw signal : Inport
  " " : Constant  Value=uPitchMin
  "   " : Constant  Value=uPitchMax
  Abs : Abs  SaturateOnIntegerOverflow=off
  Add10 : Sum  Inputs=+-
  Add12 : Sum
  Add8 : Sum
  Add9 : Sum  Inputs=+-
  Constant : Constant  Value=dirPitch
  Constant4 : Constant  Value=0
  Constant5 : Constant
  Constant6 : Constant  Value=max(uPitchMin, uPitchMax) - min(uPitchMin, uPitchMax)
  Divide : Product  Inputs=*/
  Gain : Gain  Gain=elevatorMax
  Gain1 : Gain  Gain=abs(elevatorMin)
  Gain2 : Gain  Gain=-1
  Gain6 : Gain  Gain=0.5
  Gain7 : Gain  Gain=0.5
  Gain8 : Gain  Gain=0.5
  Switch : Switch  Criteria=u2 > Threshold  Threshold=pitchDB  SaturateOnIntegerOverflow=off  InputSameDT=off
  Switch1 : Switch  SaturateOnIntegerOverflow=off  InputSameDT=off
  Switch2 : Switch  Criteria=u2 > Threshold  SaturateOnIntegerOverflow=off  InputSameDT=off
  Switch3 : Switch  Criteria=u2 > Threshold  SaturateOnIntegerOverflow=off  InputSameDT=off
  actuator deflection : Outport
  wires:
  Add9/1 -> Gain6/1
  "   "/1 -> Add9/1, Add8/1
  Add8/1 -> Gain7/1
  " "/1 -> Add8/2, Add9/2
  raw signal/1 -> Add10/1
  Gain7/1 -> Add10/2  "uMid"
  Add10/1 -> Divide/1
  Gain6/1 -> Divide/2  "uHalf"
  Switch1/1 -> actuator deflection/1
  Divide/1 -> Add12/1, Switch2/1  "y1"
  Constant5/1 -> Add12/2
  Add12/1 -> Gain8/1
  Constant6/1 -> Switch2/2
  Gain8/1 -> Switch2/3  "y2"
  Abs/1 -> Switch/2
  Constant4/1 -> Switch/3
  Switch/1 -> Gain2/1, Switch3/3
  Gain/1 -> Switch1/1
  Gain1/1 -> Switch1/3
  Gain2/1 -> Switch3/1
  Switch3/1 -> Gain1/1, Switch1/2, Gain/1
  Constant/1 -> Switch3/2
  Switch2/1 -> Switch/1, Abs/1

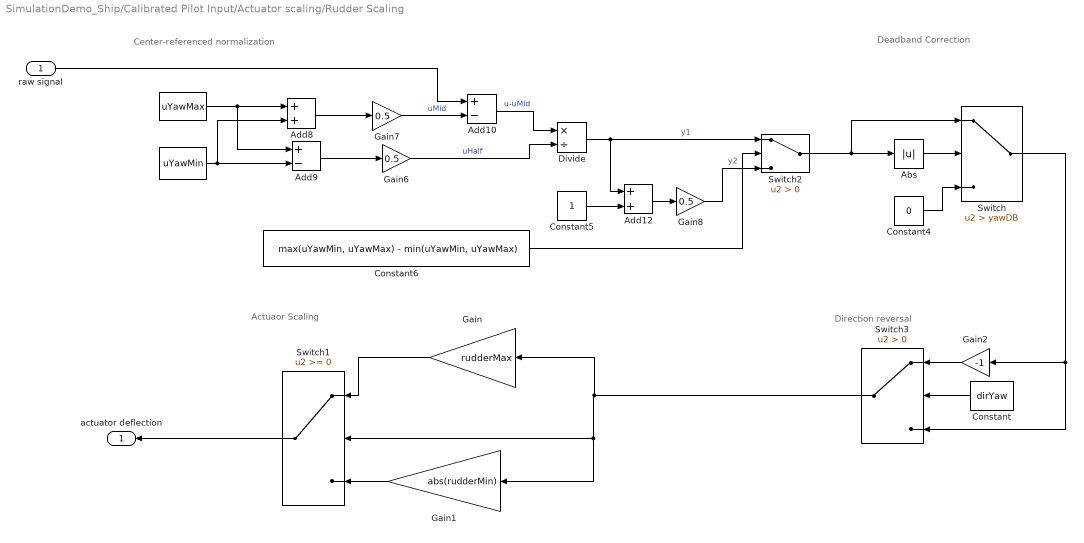
== system SimulationDemo_Ship/Calibrated Pilot Input/Actuator scaling/Rudder Scaling ==
  note: Direction reversal
  note: Center-referenced normalization
  note: Deadband Correction
  note: Actuaor Scaling
  raw signal : Inport
  " " : Constant  Value=uYawMin
  "   " : Constant  Value=uYawMax
  Abs : Abs  SaturateOnIntegerOverflow=off
  Add10 : Sum  Inputs=+-
  Add12 : Sum
  Add8 : Sum
  Add9 : Sum  Inputs=+-
  Constant : Constant  Value=dirYaw
  Constant4 : Constant  Value=0
  Constant5 : Constant
  Constant6 : Constant  Value=max(uYawMin, uYawMax) - min(uYawMin, uYawMax)
  Divide : Product  Inputs=*/
  Gain : Gain  Gain=rudderMax
  Gain1 : Gain  Gain=abs(rudderMin)
  Gain2 : Gain  Gain=-1
  Gain6 : Gain  Gain=0.5
  Gain7 : Gain  Gain=0.5
  Gain8 : Gain  Gain=0.5
  Switch : Switch  Criteria=u2 > Threshold  Threshold=yawDB  SaturateOnIntegerOverflow=off  InputSameDT=off
  Switch1 : Switch  SaturateOnIntegerOverflow=off  InputSameDT=off
  Switch2 : Switch  Criteria=u2 > Threshold  SaturateOnIntegerOverflow=off  InputSameDT=off
  Switch3 : Switch  Criteria=u2 > Threshold  SaturateOnIntegerOverflow=off  InputSameDT=off
  actuator deflection : Outport
  wires:
  Add9/1 -> Gain6/1
  "   "/1 -> Add9/1, Add8/1
  Add8/1 -> Gain7/1
  " "/1 -> Add8/2, Add9/2
  raw signal/1 -> Add10/1
  Gain7/1 -> Add10/2  "uMid"
  Add10/1 -> Divide/1  "u-uMid"
  Gain6/1 -> Divide/2  "uHalf"
  Switch1/1 -> actuator deflection/1
  Divide/1 -> Add12/1, Switch2/1  "y1"
  Constant5/1 -> Add12/2
  Add12/1 -> Gain8/1
  Constant6/1 -> Switch2/2
  Gain8/1 -> Switch2/3  "y2"
  Abs/1 -> Switch/2
  Constant4/1 -> Switch/3
  Switch/1 -> Gain2/1, Switch3/3
  Gain/1 -> Switch1/1
  Gain1/1 -> Switch1/3
  Gain2/1 -> Switch3/1
  Switch3/1 -> Gain1/1, Switch1/2, Gain/1
  Constant/1 -> Switch3/2
  Switch2/1 -> Switch/1, Abs/1

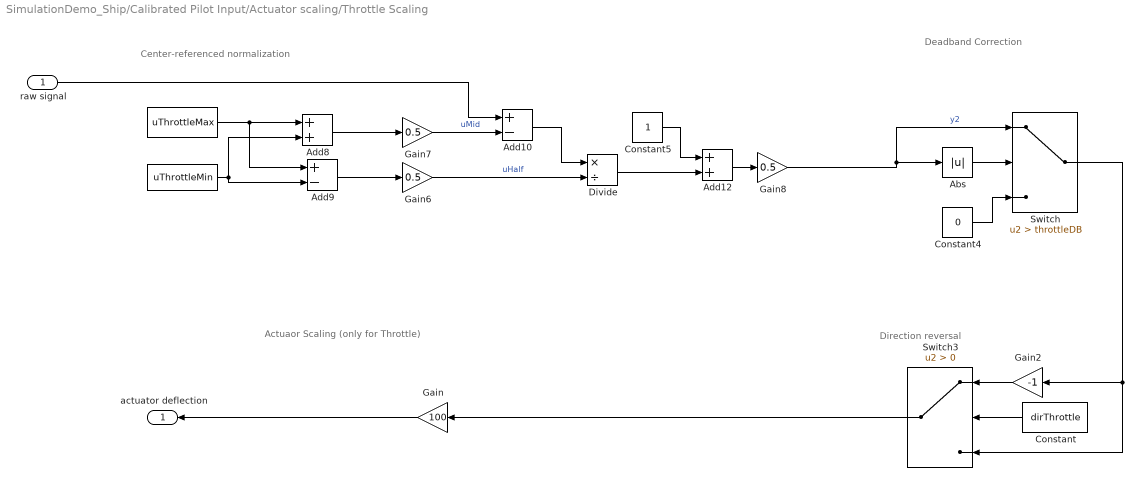
== system SimulationDemo_Ship/Calibrated Pilot Input/Actuator scaling/Throttle Scaling ==
  note: Direction reversal
  note: Center-referenced normalization
  note: Deadband Correction
  note: Actuaor Scaling (only for Throttle)
  raw signal : Inport
  " " : Constant  Value=uThrottleMin
  "   " : Constant  Value=uThrottleMax
  Abs : Abs  SaturateOnIntegerOverflow=off
  Add10 : Sum  Inputs=+-
  Add12 : Sum
  Add8 : Sum
  Add9 : Sum  Inputs=+-
  Constant : Constant  Value=dirThrottle
  Constant4 : Constant  Value=0
  Constant5 : Constant
  Divide : Product  Inputs=*/
  Gain : Gain  Gain=100
  Gain2 : Gain  Gain=-1
  Gain6 : Gain  Gain=0.5
  Gain7 : Gain  Gain=0.5
  Gain8 : Gain  Gain=0.5
  Switch : Switch  Criteria=u2 > Threshold  Threshold=throttleDB  SaturateOnIntegerOverflow=off  InputSameDT=off
  Switch3 : Switch  Criteria=u2 > Threshold  SaturateOnIntegerOverflow=off  InputSameDT=off
  actuator deflection : Outport
  wires:
  Add9/1 -> Gain6/1
  "   "/1 -> Add9/1, Add8/1
  Add8/1 -> Gain7/1
  " "/1 -> Add9/2, Add8/2
  raw signal/1 -> Add10/1
  Gain7/1 -> Add10/2  "uMid"
  Add10/1 -> Divide/1
  Gain6/1 -> Divide/2  "uHalf"
  Add12/1 -> Gain8/1
  Gain8/1 -> Switch/1, Abs/1  "y2"
  Abs/1 -> Switch/2
  Constant4/1 -> Switch/3
  Switch/1 -> Gain2/1, Switch3/3
  Gain2/1 -> Switch3/1
  Constant/1 -> Switch3/2
  Gain/1 -> actuator deflection/1
  Switch3/1 -> Gain/1
  Constant5/1 -> Add12/1
  Divide/1 -> Add12/2

== system SimulationDemo_Ship/Visualizations/Flight parameters /Scope Plot ==
  In1 : Inport
  Body : Scope  NumInputPorts=10
      settings: ActiveDisplayYMinimum=10.4194717708245  ActiveDisplayYMaximum=18.842280914352834
  Bus Selector : BusSelector  OutputSignals=Ve,Vb,Xe,Euler_angles,wb,Actuator deflections
  Bus Selector1 : BusSelector  OutputSignals=Aileron,Elevator,Rudder,Throttle
  Demux{,1,3..4} (4 alike) : Demux  Outputs=3
  Inertial : Scope  NumInputPorts=6
      settings: TimeSpan=10  ActiveDisplayYMinimum=-0.019413698996304879  ActiveDisplayYMaximum=0.0292460156648607
  Radians to Degrees1 : simulink_extras/Transformations/Radians to Degrees  Commented=through
  Radians to Degrees2 : simulink_extras/Transformations/Radians to Degrees
  wires:
  Bus Selector1/4 -> Body/10  "<Throttle>"
  Bus Selector1/3 -> Body/9  "<Rudder>"
  Bus Selector1/2 -> Body/8  "<Elevator>"
  Bus Selector1/1 -> Body/7  "<Aileron>"
  Demux1/3 -> Body/6  "r"
  Demux1/2 -> Body/5  "q"
  Demux1/1 -> Body/4  "p"
  Demux/3 -> Body/3  "w"
  Demux/2 -> Body/2  "v"
  Demux/1 -> Body/1  "u"
  Demux3/3 -> Inertial/6  "Alt"
  Demux3/2 -> Inertial/5  "Y"
  Demux3/1 -> Inertial/4  "X"
  Demux4/3 -> Inertial/3  "Psy"
  Demux4/2 -> Inertial/2  "Theta"
  Demux4/1 -> Inertial/1  "Phi"
  Bus Selector/2 -> Demux/1  "<Vb>"
  Bus Selector/6 -> Bus Selector1/1  "<Actuator deflections>"
  In1/1 -> Bus Selector/1
  Radians to Degrees2/1 -> Demux4/1  "Euler Angles"
  Bus Selector/5 -> Radians to Degrees1/1  "<wb>"
  Bus Selector/3 -> Demux3/1  "<Xe>"
  Radians to Degrees1/1 -> Demux1/1  "Euler Angles"
  Bus Selector/4 -> Radians to Degrees2/1  "<Euler_angles>"

== system SimulationDemo_Ship/Visualizations/Trajectory Visualization/3D Animation ==
  AC States : Inport
  Bus Selector : BusSelector  OutputSignals=Xe,q
  UAV_Animation : uavutilslib/UAV Animation  NumUAV=1  DynamicUAVConfig=off  UAVType=FixedWing  UAVSize=1  UAVColor=[1 0 0]  UAVTrajectoryAlpha=1  InertialZDirection=Down  RotationFormat=Quaternion  DrawMarkers=off  SampleTime=-1
  wires:
  Bus Selector/1 -> UAV_Animation/1  "<Xe>"
  Bus Selector/2 -> UAV_Animation/2  "<q>"
  AC States/1 -> Bus Selector/1

== system SimulationDemo_Ship/Visualizations/Trajectory Visualization/Unreal Engine ==
  AC States : Inport
  Bus Selector1 : BusSelector  OutputSignals=Xe,Euler_angles,Actuator deflections
  Rotation Subsystem : Subsystem
  Simulation 3D Aircraft1 : aerolibsim3d/Simulation 3D Aircraft  Priority=-1  Commented=on  Mesh=Sky Hogg  MeshPath=/MathWorksAerospaceContent/Vehicles/Aircraft/Custom/Mesh/SK_HL20.SK_HL20  MeshPathAT=/MathWorksAerospaceContent/Vehicles/Aircraft/AirTransport/Mesh/SK_AirTransport.SK_AirTransport  MeshPathGA=/MathWorksAerospaceContent/Vehicles/Aircraft/GeneralAviation/Mesh/SK_GeneralAviation.SK_GeneralAviation  AircraftColor=Red  ActorName=SimulinkVehicle3  Translation=[initial.Xe ; zeros(10, 3)]  Rotation=[0 0 initial.Heading*pi/180; zeros(10, 3)]  ScaleInputPort=Dialog  Scale=[1 1 1]  InitialScale=[1 1 1]  IsGHSensorEnabled=off  AreGHRaysVisible=off  IsOutputReshapeEnabled=off  GHRayLength=1524  GHBodyOffset=0.90  GHFrontTireRadius=0.21  GHLeftTireRadius=0.21  GHRightTireRadius=0.21  WoWSensorTolerance=0.05  LightsConfig=Automatic lights  LandingLightIntensity=300000  LandingLightConeAngle=15  CustomLeftLandingLightLocation=[0 0 0]  CustomLeftLandingLightOrientation=[0 0 0]  CustomRightLandingLightLocation=[0 0 0]  CustomRightLandingLightOrientation=[0 0 0]  TaxiLightIntensity=150000  TaxiLightConeAngle=36  CustomTaxiLightLocation=[0 0 0]  CustomTaxiLightOrientation=[0 0 0]  NavLightIntensity=500  PositionLightIntensity=500  StrobeLightIntensity=5000  WingtipStrobePeriod=1.5  WingtipStrobePulseWidth=6  TailStrobePeriod=1.5  TailStrobePulseWidth=6  BeaconLightIntensity=4000  BeaconPeriod=1.5  BeaconPulseWidth=10  SampleTime=-1  ActorType=SimulinkVehicle  ID=3  aMode=0  ActorTag=SimulinkVehicle3
  Simulation 3D Scene Configuration : sim3dlib/Simulation 3D Scene Configuration  Priority=0  ProjectFormat=Default Scenes  SceneDesc=Airport  ProjectName=C:\Program Files\MATLAB\R2025a\toolbox\shared\sim3d_projects\automotive_project_windows\UE\WindowsNoEditor\VehicleSimulation.exe  ScenePath=/Game/Maps/HwStrght  EnableOpenDRIVE=off  vehTagList={'Custom';'Scene Origin';'SimulinkVehicle2'}  vehTag=SimulinkVehicle2  AttachedCameraRelativeTranslation=[0 0 0]  FreeCameraDefaultInitialTranslation=[-6, 0, 2]  AttachedCameraRelativeRotation=[0 0 0]  FreeCameraDefaultInitialRotation=[0, -15, 0]  ViewpointName=Custom  FreeCameraInitialTranslation=[0 0 0]  ViewpointTranslation=[0 0 0]  FreeCameraInitialRotation=[0 0 0]  ViewpointRotation=[0 0 0]  OpVisEn=off  Ts=0.1  EnableWindow=on  EnableRemoteAccess=off  EnableWeather=off  SunAzimuth=90  SunAltitude=40.0  EnableGeospatialSun=off  Latitude=0  Longitude=0  Date=2023-01-01  Time=10:30:00  GeoTimeZone=-5.0  SunDaylightSaving=off  wind=1  clouds=10  EnableVolumetricClouds=off  CloudCoverage=0  CloudAltitude=6  fog=0  rain=0  RaindropsEffect=off  SnowDensity=0  EnableGeospatial=off  AccessTokenID=MyNewToken  TilesetSource=Earth terrain  UseTrueOrigin=off  OriginHeight=initial.Altitude_AGL  OriginLatitude=0  OriginLongitude=0  MapStyle=Aerial  AdditionalAssetIDs=[]  UseAdvancedSunSky=off  SolarTime=11  TimeZone=-5  Day=21  Month=9  Year=2022  UseDaylightSavingTime=on  DSTStartDay=10  DSTStartMonth=3  DSTEndDay=3  DSTEndMonth=11  DSTSwitchHour=2  sensorTag=MainCamera2  sensorId=2  sensorName=MainCamera2  mountLoc=Origin  offsetFlag=off  tmountOffset=[0, 0, 0]  rmountOffset=[0, 0, 0]  HorizontalResolution=1280  VerticalResolution=720  HorizontalFOV=60  mountPoint=[0 0 0]  mountOrientation=[0 0 0]  aMode=0  ID=2  GeoTrigger=Inactive  ViewNameList={'Custom'}  ViewTranslationList={'[0 0 0]'}  ViewRotationList={'[0 0 0]'}
      settings: AttributesFormatString=NED  LibrarySourceBlock=aerolibsim3d/Simulation 3D Scene Configuration
  Simulation 3D Sky Hogg Pack : aerolibsim3d/Simulation 3D Sky Hogg Pack  Propeller_R=on  Rudder_R=on  Elevator_R=on  Left_Aileron_R=on  Right_Aileron_R=on  Flaps_R=off  Nose_Wheel_Strut_R=off  Nose_Wheel_R=off  Left_Wheel_R=off  Right_Wheel_R=off  GeoRadioButton=NED
      settings: AttributesFormatString=NED
  wires:
  Bus Selector1/1 -> Simulation 3D Sky Hogg Pack/1  "<Xe>"
  Rotation Subsystem/1(Prop) -> Simulation 3D Sky Hogg Pack/3
  Rotation Subsystem/3(Elevator) -> Simulation 3D Sky Hogg Pack/5
  Rotation Subsystem/4(Left aileron) -> Simulation 3D Sky Hogg Pack/6
  AC States/1 -> Bus Selector1/1
  Simulation 3D Sky Hogg Pack/2 -> Simulation 3D Aircraft1/2
  Simulation 3D Sky Hogg Pack/1 -> Simulation 3D Aircraft1/1
  Rotation Subsystem/2(Rudder) -> Simulation 3D Sky Hogg Pack/4
  Rotation Subsystem/5(Right aileron) -> Simulation 3D Sky Hogg Pack/7
  Bus Selector1/2 -> Simulation 3D Sky Hogg Pack/2  "<Euler_angles>"
  Bus Selector1/3 -> Rotation Subsystem/1(Pilot)  "<Actuator deflections>"

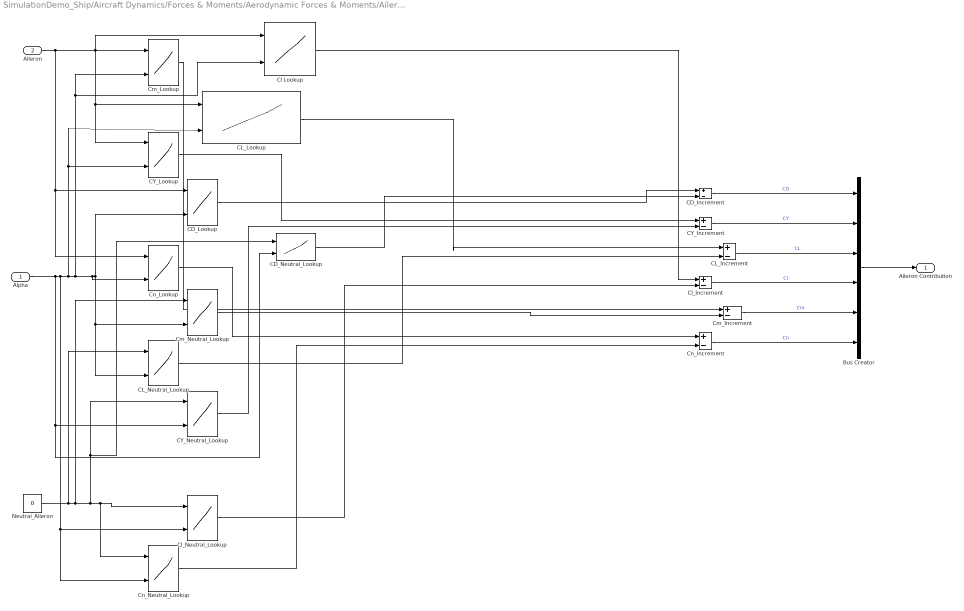
== system SimulationDemo_Ship/Aircraft Dynamics/Forces & Moments/Aerodynamic Forces & Moments/Aileron Contribution ==
  Alpha : Inport
  Aileron : Inport  Port=2
  Bus Creator : BusCreator  Inputs=6
  CD_Increment : Sum  Inputs=+-
  CD_Lookup : Lookup_n-D  BreakpointsForDimension1=aeroData.aileronData.ControlDeflections  BreakpointsForDimension2=aeroData.aileronData.Alpha  Table=aeroData.aileronData.CD
      settings: InputPortMap=u0,u1
  CD_Neutral_Lookup : Lookup_n-D  BreakpointsForDimension1=aeroData.aileronData.ControlDeflections  BreakpointsForDimension2=aeroData.aileronData.Alpha  Table=aeroData.aileronData.CD
      settings: InputPortMap=u0,u1
  CL_Increment : Sum  Inputs=+-
  CL_Lookup : Lookup_n-D  BreakpointsForDimension1=aeroData.aileronData.ControlDeflections  BreakpointsForDimension2=aeroData.aileronData.Alpha  Table=aeroData.aileronData.CL
      settings: InputPortMap=u0,u1
  CL_Neutral_Lookup : Lookup_n-D  BreakpointsForDimension1=aeroData.aileronData.ControlDeflections  BreakpointsForDimension2=aeroData.aileronData.Alpha  Table=aeroData.aileronData.CL
      settings: InputPortMap=u0,u1
  CY_Increment : Sum  Inputs=+-
  CY_Lookup : Lookup_n-D  BreakpointsForDimension1=aeroData.aileronData.ControlDeflections  BreakpointsForDimension2=aeroData.aileronData.Alpha  Table=aeroData.aileronData.CY
      settings: InputPortMap=u0,u1
  CY_Neutral_Lookup : Lookup_n-D  BreakpointsForDimension1=aeroData.aileronData.ControlDeflections  BreakpointsForDimension2=aeroData.aileronData.Alpha  Table=aeroData.aileronData.CY
      settings: InputPortMap=u0,u1
  "Cl Lookup " : Lookup_n-D  BreakpointsForDimension1=aeroData.aileronData.ControlDeflections  BreakpointsForDimension2=aeroData.aileronData.Alpha  Table=aeroData.aileronData.Cl  InternalRulePriority=Speed  RndMeth=Simplest
      settings: InputPortMap=u0,u1
  Cl_Increment : Sum  Inputs=+-
  Cl_Neutral_Lookup : Lookup_n-D  BreakpointsForDimension1=aeroData.aileronData.ControlDeflections  BreakpointsForDimension2=aeroData.aileronData.Alpha  Table=aeroData.aileronData.Cl
      settings: InputPortMap=u0,u1
  Cm_Increment : Sum  Inputs=+-
  Cm_Lookup : Lookup_n-D  BreakpointsForDimension1=aeroData.aileronData.ControlDeflections  BreakpointsForDimension2=aeroData.aileronData.Alpha  Table=aeroData.aileronData.Cm
      settings: InputPortMap=u0,u1
  Cm_Neutral_Lookup : Lookup_n-D  BreakpointsForDimension1=aeroData.aileronData.ControlDeflections  BreakpointsForDimension2=aeroData.aileronData.Alpha  Table=aeroData.aileronData.Cm
      settings: InputPortMap=u0,u1
  Cn_Increment : Sum  Inputs=+-
  Cn_Lookup : Lookup_n-D  BreakpointsForDimension1=aeroData.aileronData.ControlDeflections  BreakpointsForDimension2=aeroData.aileronData.Alpha  Table=aeroData.aileronData.Cn
      settings: InputPortMap=u0,u1
  Cn_Neutral_Lookup : Lookup_n-D  BreakpointsForDimension1=aeroData.aileronData.ControlDeflections  BreakpointsForDimension2=aeroData.aileronData.Alpha  Table=aeroData.aileronData.Cn
      settings: InputPortMap=u0,u1
  Neutral_Aileron : Constant  Value=0
  Aileron Contribution : Outport
  wires:
  Cn_Increment/1 -> Bus Creator/6  "Cn"
  Cn_Neutral_Lookup/1 -> Cn_Increment/2
  Cn_Lookup/1 -> Cn_Increment/1
  Cm_Increment/1 -> Bus Creator/5  "Cm"
  Cm_Neutral_Lookup/1 -> Cm_Increment/2
  Cm_Lookup/1 -> Cm_Increment/1
  CL_Increment/1 -> Bus Creator/3  "CL"
  CL_Neutral_Lookup/1 -> CL_Increment/2
  CL_Lookup/1 -> CL_Increment/1
  CY_Increment/1 -> Bus Creator/2  "CY"
  CY_Neutral_Lookup/1 -> CY_Increment/2
  CY_Lookup/1 -> CY_Increment/1
  CD_Increment/1 -> Bus Creator/1  "CD"
  CD_Neutral_Lookup/1 -> CD_Increment/2
  CD_Lookup/1 -> CD_Increment/1
  Aileron/1 -> Cn_Lookup/1, CD_Lookup/1, CY_Lookup/1, CL_Lookup/1, "Cl Lookup "/1, Cm_Lookup/1
  Alpha/1 -> CD_Neutral_Lookup/2, CY_Neutral_Lookup/2, Cl_Neutral_Lookup/2, Cn_Neutral_Lookup/2, CL_Neutral_Lookup/2, Cm_Neutral_Lookup/2, CD_Lookup/2, Cn_Lookup/2, "Cl Lookup "/2, Cm_Lookup/2, CY_Lookup/2, CL_Lookup/2
  Neutral_Aileron/1 -> Cl_Neutral_Lookup/1, Cn_Neutral_Lookup/1, CD_Neutral_Lookup/1, CY_Neutral_Lookup/1, Cm_Neutral_Lookup/1, CL_Neutral_Lookup/1
  "Cl Lookup "/1 -> Cl_Increment/1
  Cl_Neutral_Lookup/1 -> Cl_Increment/2
  Cl_Increment/1 -> Bus Creator/4  "Cl"
  Bus Creator/1 -> Aileron Contribution/1

== system SimulationDemo_Ship/Aircraft Dynamics/Forces & Moments/Aerodynamic Forces & Moments/Beta_Protection ==
  beta : Inport
  Vrel : Inport  Port=2
  BetaLimit : Saturate  UpperLimit=aeroData.validBetaRange_deg(2)  LowerLimit=aeroData.validBetaRange_deg(1)
  Beta_Effective : Product
  Beta_Gate_Limit : Saturate  UpperLimit=1  LowerLimit=0
  Beta_Gate_Slope : Gain  Gain=1/(flightProtection.BetaGateFullU_mps-flightProtection.BetaGateStartU_mps)
  Beta_Gate_Start_U : Constant  Value=flightProtection.BetaGateStartU_mps
  Split_Vrel : Demux  Outputs=3
  Unused_vrel : Terminator
  Unused_wrel : Terminator
  Urel_Minus_Gate_Start : Sum  Inputs=+-
  beta_effective : Outport
  wires:
  Split_Vrel/3 -> Unused_wrel/1
  Split_Vrel/2 -> Unused_vrel/1
  Beta_Effective/1 -> beta_effective/1
  Beta_Gate_Limit/1 -> Beta_Effective/2
  Beta_Gate_Slope/1 -> Beta_Gate_Limit/1
  Urel_Minus_Gate_Start/1 -> Beta_Gate_Slope/1
  Beta_Gate_Start_U/1 -> Urel_Minus_Gate_Start/2
  Split_Vrel/1 -> Urel_Minus_Gate_Start/1
  Vrel/1 -> Split_Vrel/1
  BetaLimit/1 -> Beta_Effective/1
  beta/1 -> BetaLimit/1

== system SimulationDemo_Ship/Aircraft Dynamics/Forces & Moments/Aerodynamic Forces & Moments/Damping rate coefficients ==
  beta : Inport
  p,q,r : Inport  Port=2  Unit=rad/second
  V_TAS : Inport  Port=3  Unit=m/second
  Beta_Deg_to_Rad : Gain  Gain=pi/180
  Bus Creator : BusCreator  Inputs=6
  CL_q : Product  Inputs=**
  CLq : Constant  Value=aeroData.stabilityDerivatives.CLq
  CY_Derivative_Sum : Sum  Inputs=+++
  CY_beta : Product  Inputs=**
  CY_p : Product  Inputs=**
  CY_r : Product  Inputs=**
  CYb : Constant  Value=aeroData.stabilityDerivatives.CYb
  CYp : Constant  Value=aeroData.stabilityDerivatives.CYp
  CYr : Constant  Value=aeroData.stabilityDerivatives.CYr
  Cl : Subsystem
  Cm : Subsystem
  Cn : Subsystem
  Non Dimensionalize p,q,r : Subsystem
  Zero_CD_Derivative : Constant  Value=0
  Damping rate contributions : Outport
  wires:
  V_TAS/1 -> Non Dimensionalize p,q,r/2(V_TAS)
  p,q,r/1 -> Non Dimensionalize p,q,r/1(p,q,r)
  CL_q/1 -> Bus Creator/3  "CL_rate"
  beta/1 -> Beta_Deg_to_Rad/1
  Cl/1(Cl_damp) -> Bus Creator/4  "Cl_damp"
  CYr/1 -> CY_r/1
  CYb/1 -> CY_beta/1
  Non Dimensionalize p,q,r/2(q_nd) -> CL_q/2, Cm/1(q_nd)
  CLq/1 -> CL_q/1
  CYp/1 -> CY_p/1
  Beta_Deg_to_Rad/1 -> CY_beta/2, Cn/2(beta), Cl/2(beta)
  Non Dimensionalize p,q,r/1(p_nd) -> Cn/1(p_nd), CY_p/2, Cl/1(p_nd)
  Non Dimensionalize p,q,r/3(r_nd) -> Cn/3(r_nd), CY_r/2, Cl/3(r_nd)
  Zero_CD_Derivative/1 -> Bus Creator/1  "CD_rate"
  CY_beta/1 -> CY_Derivative_Sum/1
  CY_p/1 -> CY_Derivative_Sum/2
  CY_r/1 -> CY_Derivative_Sum/3
  Cm/1(Cm_damp) -> Bus Creator/5  "Cm_damp"
  Cn/1(Cn_damp) -> Bus Creator/6  "Cn_damp"
  CY_Derivative_Sum/1 -> Bus Creator/2  "CY_rate"
  Bus Creator/1 -> Damping rate contributions/1
